simulink model "dead1"  (Simulink 3.00)
settings: Solver=ode45  SolverMode=SingleTasking  StartTime=0.0  StopTime=40  MaxStep=0.010  RelTol=1e-3  AbsTol=1e-3
undefined symbols (not defined in the file or in its folder): dz
settings Model: TimeSaveName=t  SaveOutput=off

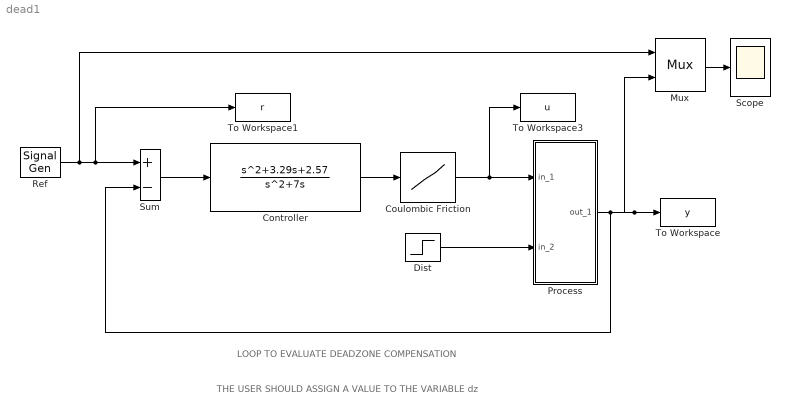
== system dead1 ==
  note: LOOP TO EVALUATE DEADZONE COMPENSATION
  note: THE USER SHOULD ASSIGN A VALUE TO THE VARIABLE dz
  Controller : TransferFcn  Numerator=[1 3.29 2.57]  Denominator=[1 7 0]
  Coulombic Friction : Lookup  InputValues=[-1,0,0,1]  OutputValues=[-gain-ini -ini ini gain+ini]  mask(Coulombic Friction){ini=dz, gain=1}
      mask prompts: ini "Offset discontinuity at zero:"
      mask help:
      | Coulombic Friction
      | y = sign(x) * (Gain * abs(x) + Offset)
      mask init:
      | x=max(ini,gain+ini);
      mask Help: This block has a discontinuity\nat zero and a linear gain afterward.\ny= sign(x)*(Gain*abs(x)+Offset)
      mask Display: plot([-1 0 0 1],[-gain-ini, -ini, ini, gain+ini],[-1 1],[0 0],[0 0],[-x,x])
  Dist : Step  Time=10  Before=0  After=1  SampleTime=0
  Mux : Mux  Inputs=2
      settings: DisplayOption=none
  "Process " : Subsystem
      mask Type: Plant
      mask Display: disp('PLANT')
  Ref : SignalGenerator  WaveForm=square  Amplitude=1.000000  Frequency=0.100000  Units=rad/sec
  Scope : Scope
      settings: TickLabels=on  TimeRange=40.000000  YMin=-2  YMax=2  SaveToWorkspace=off  SaveName=ScopeData  DataFormat=Matrix
  Sum : Sum  Inputs=+-  SaturateOnIntegerOverflow=on
  To Workspace : ToWorkspace  VariableName=y  SampleTime=0  SaveFormat=Matrix
      settings: Buffer=10000
  To Workspace1 : ToWorkspace  VariableName=r  SampleTime=0  SaveFormat=Matrix
      settings: Buffer=10000
  To Workspace3 : ToWorkspace  VariableName=u  SampleTime=0  SaveFormat=Matrix
      settings: Buffer=10000
  wires:
  Sum/1 -> Controller/1
  Controller/1 -> Coulombic Friction/1
  "Process "/1(out_1) -> Sum/2, To Workspace/1, Mux/2
  Dist/1 -> "Process "/2(in_2)
  Coulombic Friction/1 -> "Process "/1(in_1), To Workspace3/1
  Mux/1 -> Scope/1
  Ref/1 -> Sum/1, To Workspace1/1, Mux/1

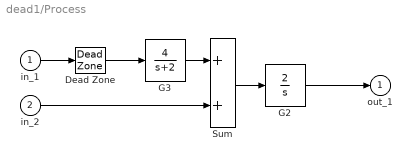
== system dead1/Process  ==
  in_1 : Inport  Port=1  PortWidth=-1  SampleTime=-1  DataType=auto
      settings: SignalType=auto
  in_2 : Inport  Port=2  PortWidth=-1  SampleTime=-1  DataType=auto
      settings: SignalType=auto
  Dead Zone : DeadZone  LowerValue=-dz  UpperValue=dz
  G2 : TransferFcn  Numerator=[2]  Denominator="[1  0]"
  G3 : TransferFcn  Numerator=4  Denominator="[1  2]"
  Sum : Sum  Inputs=++  SaturateOnIntegerOverflow=on
  out_1 : Outport  Port=1  InitialOutput=0
  wires:
  G2/1 -> out_1/1
  in_1/1 -> Dead Zone/1
  Dead Zone/1 -> G3/1
  Sum/1 -> G2/1
  G3/1 -> Sum/1
  in_2/1 -> Sum/2
